simulink model "open_loop_motor"  (R2023b)
settings: Solver=ode45  StartTime=0.0  StopTime=20  RelTol=1e-3  EnableMultiTasking=on
settings Model: Creator=yoany  LastModifiedBy=yoany
settings SolverCC: AlgebraicLoopSolver=TrustRegion
settings DataIOCC: LimitDataPoints=on  SaveFormat=Array  SignalLoggingSaveFormat=ModelDataLogs  ReturnWorkspaceOutputs=off
settings OptimizationCC: BooleanDataType=off  LifeSpan=inf
settings DebuggingCC: SaveWithParameterizedLinksMsg=none  UnderspecifiedInitializationDetection=Classic  MergeDetectMultiDrivingBlocksExec=none  SignalResolutionControl=TryResolveAllWithWarning  MultiTaskDSMMsg=warning  MultiTaskCondExecSysMsg=none  UnconnectedInputMsg=warning  UnconnectedOutputMsg=warning  UnconnectedLineMsg=warning  SFUnexpectedBacktrackingDiag=warning  SFNoUnconditionalDefaultTransitionDiag=warning  ArithmeticOperatorsInVariantConditions=warning
settings HardwareCC: TargetUnknown=on
settings ModelReferenceCC: EnableRefExpFcnMdlSchedulingChecks=on  PropagateSignalLabelsOutOfModel=off
settings SFSimCC: SimUseLocalCustomCode=off  CustomCodeUndefinedFunction=UseInterfaceOnly
settings RTWCC: RTWUseLocalCustomCode=off
settings CodeAppCC: StateflowObjectComments=on
settings GRTTargetCC: TargetLangStandard=C89/C90 (ANSI)  CombineOutputUpdateFcns=off  GRTInterface=on
settings ConfigComp: CovMetricSettings=dw  CovSaveCumulativeToWorkspaceVar=on  CovSaveSingleToWorkspaceVar=on  CovExternalEMLEnable=off

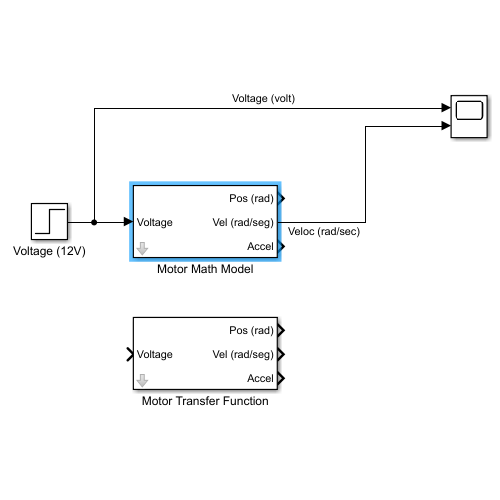
[thumbnail: Simulink's stored preview of the top-level diagram]
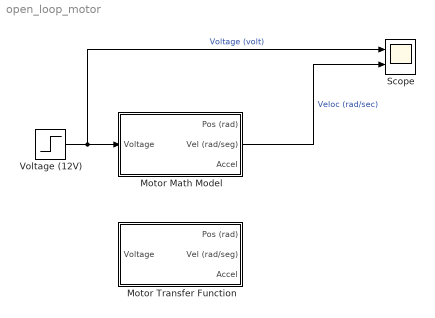
== system open_loop_motor ==
  Motor Math Model : Subsystem  mask{Ra=3.4, La=0.0015, J=0.000400955, F=0.002235795, K=0.2335, Kb=0.2335, Re=1/90}
  Motor Transfer Function : Subsystem  mask{Ra=3.4, La=0.0015, J=0.000400955, F=0.002235795, K=0.2335, Kb=0.2335, Re=1/90}
  Scope : Scope  NumInputPorts=2
  Voltage (12V) : Step  After=12  SampleTime=0
  wires:
  Motor Math Model/2(Vel (rad/seg)) -> Scope/2  "Veloc (rad/sec)"
  Voltage (12V)/1 -> Scope/1, Motor Math Model/1(Voltage)  "Voltage (volt)"

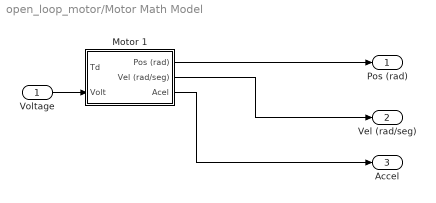
== system open_loop_motor/Motor Math Model ==
  Voltage : Inport
  Motor 1 : Subsystem  mask{Ra=Ra, La=La, J=J, F=F, K=K, Kb=Kb, Re=Re}
  Pos (rad) : Outport
  Vel (rad/seg) : Outport  Port=2
  Accel : Outport  Port=3
  wires:
  Voltage/1 -> Motor 1/2(Volt)
  Motor 1/1(Pos (rad)) -> Pos (rad)/1
  Motor 1/2(Vel (rad/seg)) -> Vel (rad/seg)/1
  Motor 1/3(Acel) -> Accel/1

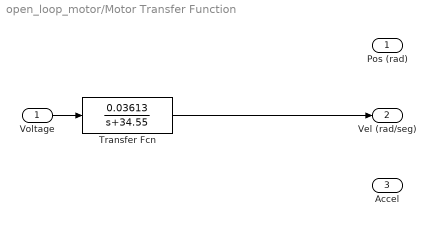
== system open_loop_motor/Motor Transfer Function ==
  Voltage : Inport
  Transfer Fcn : TransferFcn  Numerator=[0.03613]  Denominator=[1 34.55]
  Pos (rad) : Outport
  Vel (rad/seg) : Outport  Port=2
  Accel : Outport  Port=3
  wires:
  Voltage/1 -> Transfer Fcn/1
  Transfer Fcn/1 -> Vel (rad/seg)/1

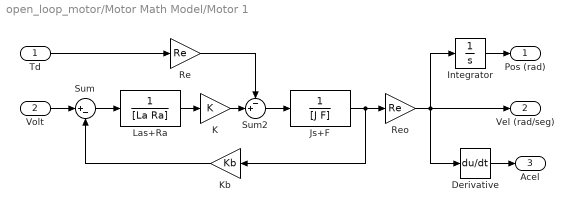
== system open_loop_motor/Motor Math Model/Motor 1 ==
  Td : Inport
  Volt : Inport  Port=2
  Derivative : Derivative
  Integrator : Integrator
  Js+F : TransferFcn  Denominator=[J F]
  K : Gain  Gain=K  SaturateOnIntegerOverflow=on  OutDataTypeStr=Inherit: Same as input  ParamDataTypeStr=Inherit: Same as input
  Kb : Gain  Gain=Kb  SaturateOnIntegerOverflow=on  OutDataTypeStr=Inherit: Same as input  ParamDataTypeStr=Inherit: Same as input
  Las+Ra : TransferFcn  Denominator=[La Ra]
  Re : Gain  Gain=Re  SaturateOnIntegerOverflow=on  OutDataTypeStr=Inherit: Same as input  ParamDataTypeStr=Inherit: Same as input
  Reo : Gain  Gain=Re  SaturateOnIntegerOverflow=on  OutDataTypeStr=Inherit: Same as input  ParamDataTypeStr=Inherit: Same as input
  Sum : Sum  Inputs=|+-  InputSameDT=on  SaturateOnIntegerOverflow=on  OutDataTypeStr=Inherit: Same as first input
  Sum2 : Sum  Inputs=-+|  InputSameDT=on  SaturateOnIntegerOverflow=on  OutDataTypeStr=Inherit: Same as first input
  Pos (rad) : Outport
  Vel (rad/seg) : Outport  Port=2
  Acel : Outport  Port=3
  wires:
  Derivative/1 -> Acel/1
  Integrator/1 -> Pos (rad)/1
  Reo/1 -> Derivative/1, Integrator/1, Vel (rad/seg)/1
  Td/1 -> Re/1
  Volt/1 -> Sum/1
  Re/1 -> Sum2/1
  K/1 -> Sum2/2
  Las+Ra/1 -> K/1
  Js+F/1 -> Reo/1, Kb/1
  Sum2/1 -> Js+F/1
  Kb/1 -> Sum/2
  Sum/1 -> Las+Ra/1
